simulink model "controller"  (R2018b)
settings: Solver=FixedStepDiscrete  StartTime=0.0  StopTime=10.0  RelTol=1e-3
settings Model: DataTypeOverride=Off  Creator=wasee  LastModifiedBy=wasee
settings DataIOCC: SaveOutput=off  SaveTime=off
settings OptimizationCC: BlockReduction=off  ConditionallyExecuteInputs=off  DefaultParameterBehavior=Inlined
settings DebuggingCC: AlgebraicLoopMsg=error  InheritedTsInSrcMsg=none  SingleTaskRateTransMsg=error
settings HardwareCC: ProdBitPerPointer=32  ProdBitPerSizeT=32  ProdBitPerPtrDiffT=32  ProdLargestAtomicFloat=None  ProdIntDivRoundTo=Undefined  ProdEndianess=Unspecified  ProdWordSize=32  ProdHWDeviceType=ASIC/FPGA->ASIC/FPGA  TargetBitPerPointer=64  TargetBitPerSizeT=64  TargetBitPerPtrDiffT=64  TargetLongLongMode=on  TargetIntDivRoundTo=Zero  TargetEndianess=LittleEndian  TargetWordSize=64  TargetHWDeviceType=Custom Processor->MATLAB Host Computer  ProdEqTarget=off

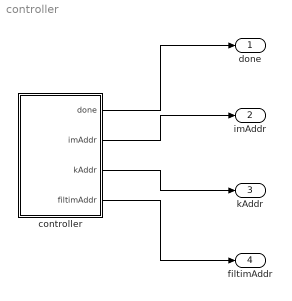
== system controller ==
  controller : Subsystem
  done : Outport  OutDataTypeStr=fixdt(0, 1, 0)
  imAddr : Outport  Port=2  OutDataTypeStr=uint16
  kAddr : Outport  Port=3  OutDataTypeStr=uint16
  filtimAddr : Outport  Port=4  OutDataTypeStr=uint16
  wires:
  controller/1(done) -> done/1
  controller/2(imAddr) -> imAddr/1
  controller/3(kAddr) -> kAddr/1
  controller/4(filtimAddr) -> filtimAddr/1

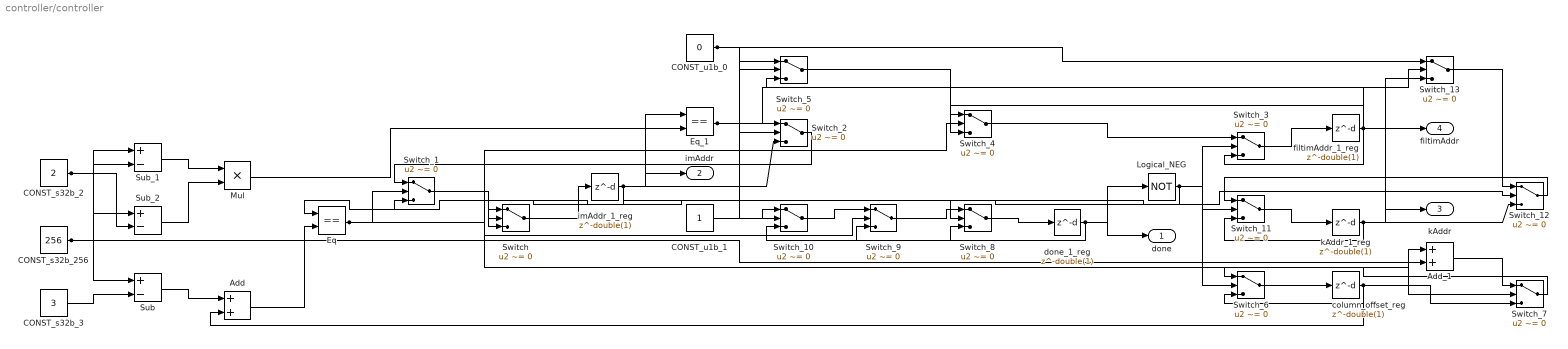
== system controller/controller ==
  Add : Sum  SampleTime=-1  OutDataTypeStr=Inherit: Same as first input
  Add_1 : Sum  AccumDataTypeStr=uint8  OutDataTypeStr=uint8  SampleTime=-1
  CONST_s32b_2 : Constant  Value=2  OutDataTypeStr=int32  SampleTime=-1
  CONST_s32b_256 : Constant  Value=256  OutDataTypeStr=int32  SampleTime=-1
  CONST_s32b_3 : Constant  Value=3  OutDataTypeStr=int32  SampleTime=-1
  CONST_u1b_0 : Constant  Value=0  OutDataTypeStr=fixdt(0, 1, 0)  SampleTime=-1
  CONST_u1b_1 : Constant  OutDataTypeStr=fixdt(0, 1, 0)  SampleTime=-1
  Eq : RelationalOperator  Operator===  OutDataTypeStr=boolean  SampleTime=-1  RndMeth=Nearest  InputSameDT=on
  Eq_1 : RelationalOperator  Operator===  OutDataTypeStr=boolean  SampleTime=-1  RndMeth=Nearest  InputSameDT=on
  Logical_NEG : Logic  Operator=NOT  Inputs=1  AllPortsSameDT=off  OutDataTypeStr=fixdt(0, 1, 0)  SampleTime=-1
  Mul : Product  Inputs=**  SampleTime=-1  OutDataTypeStr=Inherit: Same as first input
  Sub : Sum  Inputs=+-  SampleTime=-1  OutDataTypeStr=Inherit: Same as first input
  Sub_1 : Sum  Inputs=+-  SampleTime=-1  OutDataTypeStr=Inherit: Same as first input
  Sub_2 : Sum  Inputs=+-  SampleTime=-1  OutDataTypeStr=Inherit: Same as first input
  Switch : Switch  Criteria=u2 ~= 0  Threshold=double(0)  OutDataTypeStr=uint16  SampleTime=-1
  Switch_{1..5,11..13} (8 alike) : Switch  Criteria=u2 ~= 0  Threshold=double(0)  OutDataTypeStr=uint16  SampleTime=-1
  Switch_10 : Switch  Criteria=u2 ~= 0  Threshold=double(0)  OutDataTypeStr=fixdt(0, 1, 0)  SampleTime=-1
  Switch_6 : Switch  Criteria=u2 ~= 0  Threshold=double(0)  OutDataTypeStr=uint8  SampleTime=-1
  Switch_7 : Switch  Criteria=u2 ~= 0  Threshold=double(0)  OutDataTypeStr=uint8  SampleTime=-1
  Switch_8 : Switch  Criteria=u2 ~= 0  Threshold=double(0)  OutDataTypeStr=fixdt(0, 1, 0)  SampleTime=-1
  Switch_9 : Switch  Criteria=u2 ~= 0  Threshold=double(0)  OutDataTypeStr=fixdt(0, 1, 0)  SampleTime=-1
  column_offset_reg : Delay  DelayLength=double(1)  InitialCondition=0  InputProcessing=Inherited  SampleTime=-1
  done_1_reg : Delay  DelayLength=double(1)  InitialCondition=0  InputProcessing=Inherited  SampleTime=-1
  filtimAddr_1_reg : Delay  DelayLength=double(1)  InitialCondition=0  InputProcessing=Inherited  SampleTime=-1
  imAddr_1_reg : Delay  DelayLength=double(1)  InitialCondition=0  InputProcessing=Inherited  SampleTime=-1
  kAddr_1_reg : Delay  DelayLength=double(1)  InitialCondition=0  InputProcessing=Inherited  SampleTime=-1
  done : Outport  OutDataTypeStr=fixdt(0, 1, 0)
  imAddr : Outport  Port=2  OutDataTypeStr=uint16
  kAddr : Outport  Port=3  OutDataTypeStr=uint16
  filtimAddr : Outport  Port=4  OutDataTypeStr=uint16
  wires:
  CONST_s32b_256/1 -> Add_1/2, Sub_2/1, Sub_1/1, Sub/1
  CONST_s32b_3/1 -> Sub/2
  done_1_reg/1 -> Switch_10/3, Switch_9/3, Switch_8/3, Logical_NEG/1, done/1
  Switch_8/1 -> done_1_reg/1
  CONST_u1b_0/1 -> Switch_13/1, Switch_5/1, Switch_2/1
  imAddr_1_reg/1 -> Eq_1/1, Switch_2/3, Eq/1, Switch_1/3, Switch/3, imAddr/1
  Switch/1 -> imAddr_1_reg/1
  kAddr_1_reg/1 -> Switch_13/3, Switch_12/3, Switch_11/3, kAddr/1
  Switch_11/1 -> kAddr_1_reg/1
  filtimAddr_1_reg/1 -> Switch_5/3, Switch_4/3, Switch_3/3, filtimAddr/1
  Switch_3/1 -> filtimAddr_1_reg/1
  Switch_6/1 -> column_offset_reg/1
  column_offset_reg/1 -> Add_1/1, Switch_7/3, Switch_6/3, Add/2
  Logical_NEG/1 -> Switch_11/2, Switch_8/2, Switch_6/2, Switch_3/2, Switch/2
  Switch_1/1 -> Switch/1
  Eq/1 -> Switch_12/2, Switch_9/2, Switch_7/2, Switch_4/2, Switch_1/2
  Add/1 -> Eq/2
  Sub/1 -> Add/1
  Switch_2/1 -> Switch_1/1
  Eq_1/1 -> Switch_13/2, Switch_10/2, Switch_5/2, Switch_2/2
  Mul/1 -> Eq_1/2
  Sub_1/1 -> Mul/1
  CONST_s32b_2/1 -> Sub_2/2, Sub_1/2
  Sub_2/1 -> Mul/2
  Switch_4/1 -> Switch_3/1
  Switch_5/1 -> Switch_4/1
  Switch_7/1 -> Switch_6/1
  Add_1/1 -> Switch_7/1
  Switch_9/1 -> Switch_8/1
  Switch_10/1 -> Switch_9/1
  CONST_u1b_1/1 -> Switch_10/1
  Switch_12/1 -> Switch_11/1
  Switch_13/1 -> Switch_12/1
